simulink model "sampleModel1516"  (R2023a)
settings: Solver=VariableStepAuto  StartTime=0.0  StopTime=10.0  RelTol=1e-3
libraries: hdlsllib x5, simulink x1
settings Model: Creator=user1  LastModifiedBy=user1

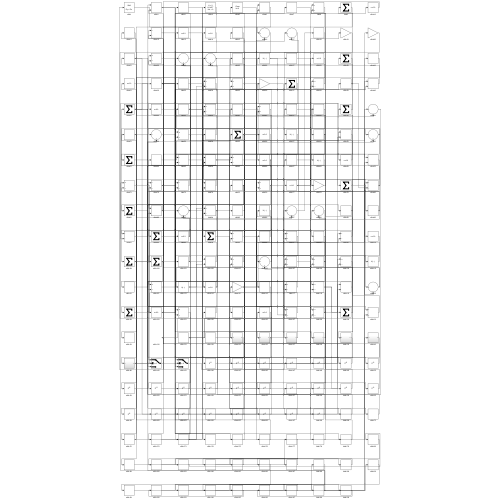
[thumbnail: Simulink's stored preview of the top-level diagram]
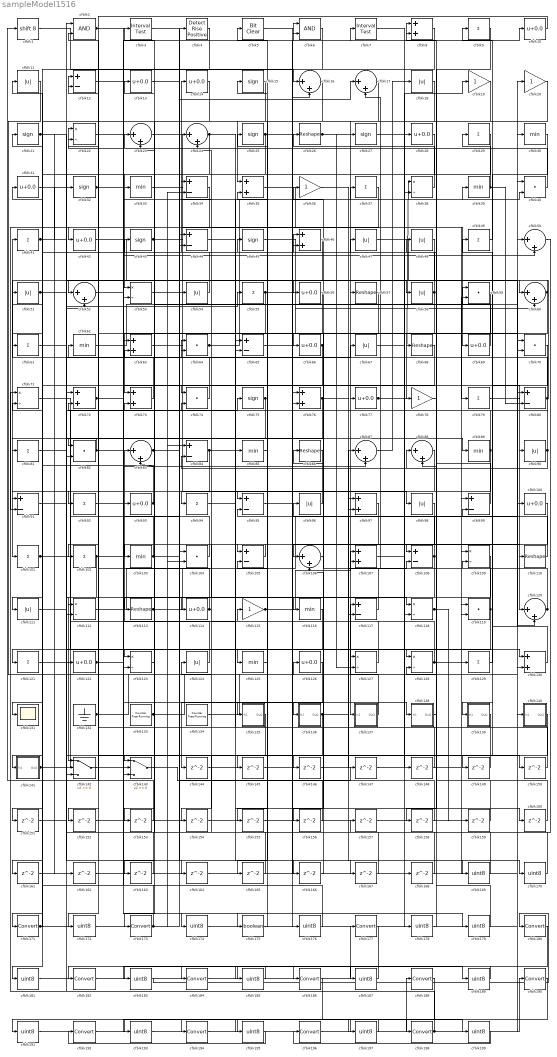
== system sampleModel1516 ==
  cfblk1 : ArithShift  BitShiftNumber=8
  cfblk{10,13..14,28,31,42,56,66,69,77,93,100,114,122,126} (15 alike) : Bias  Bias=0.0  SaturateOnIntegerOverflow=off
  cfblk{9,29,37,41,49,55,61,79,81,92,94,101..102,121,129} (15 alike) : Sum  Inputs=+
  cfblk{30,33,39,62,85,89,103,116,125} (9 alike) : MinMax
  cfblk{40,59,64,70,74,82,104,119} (8 alike) : DotProduct  OutDataTypeStr=Inherit: Inherit via internal rule
  cfblk{12,34,44,65,80,84,91,95,99,105,108,117} (12 alike) : Sum  Inputs=+-
  cfblk{16..17,23..24,50,52,60,83,87..88,106,120} (12 alike) : Sum  Inputs=|++
  cfblk{8,35,46,63,72..73,76,97,107,130} (10 alike) : Sum
  cfblk{22,38,53,71,109,112,118,123,127..128} (10 alike) : Product  Inputs=*/  RndMeth=Zero  SaturateOnIntegerOverflow=on
  cfblk{11,18,47..48,51,54,58,67,90,96,98,111,124} (13 alike) : Abs  SaturateOnIntegerOverflow=off
  cfblk{26,57,68,86,110,113} (6 alike) : Reshape
  cfblk{19..20,36,78,115} (5 alike) : Gain
  cfblk131 : Scope
  cfblk132 : Ground
  cfblk133 : hdlsllib/Sources/Counter Free-Running  NumBits=16  tsamp=-1
  cfblk134 : hdlsllib/Sources/Counter Free-Running  NumBits=16  tsamp=-1
  cfblk135 : Subsystem
      settings: LibrarySourceBlock=|
      | hdlsllib/Ports &
      | Subsystems/Subsystem
  cfblk136 : Subsystem
      settings: LibrarySourceBlock=|
      | hdlsllib/Ports &
      | Subsystems/Subsystem
  cfblk137 : Subsystem
      settings: LibrarySourceBlock=|
      | hdlsllib/Ports &
      | Subsystems/Subsystem
  cfblk138 : Subsystem
      settings: LibrarySourceBlock=|
      | hdlsllib/Ports &
      | Subsystems/Subsystem
  cfblk139 : Subsystem
      settings: LibrarySourceBlock=|
      | hdlsllib/Ports &
      | Subsystems/Subsystem
  cfblk140 : Subsystem
      settings: LibrarySourceBlock=|
      | hdlsllib/Ports &
      | Subsystems/Subsystem
  cfblk141 : Subsystem
      settings: LibrarySourceBlock=|
      | hdlsllib/Ports &
      | Subsystems/Subsystem
  cfblk142 : Switch  SaturateOnIntegerOverflow=off  InputSameDT=off
  cfblk143 : Switch  SaturateOnIntegerOverflow=off  InputSameDT=off
  cfblk{144..168} (25 alike) : Delay  SampleTime=1
  cfblk{15,21,25,27,32,43,45,75} (8 alike) : Signum
  cfblk{169..170,172,174,176,178..179,181,183,185,187,189,191,193,195,197,199} (17 alike) : DataTypeConversion  OutDataTypeStr=uint8  SaturateOnIntegerOverflow=off  RndMeth=Floor
  cfblk{171,173,177,180,182,184,186,188,190,192,194,196,198} (13 alike) : DataTypeConversion  SaturateOnIntegerOverflow=off  RndMeth=Floor
  cfblk175 : DataTypeConversion  OutDataTypeStr=boolean  SaturateOnIntegerOverflow=off  RndMeth=Floor
  cfblk2 : Logic  AllPortsSameDT=off  OutDataTypeStr=boolean
  cfblk3 : hdlsllib/Logic and Bit Operations/Interval Test  IntervalClosedRight=on  uplimit=0.5  IntervalClosedLeft=on  lowlimit=-0.5  OutDataTypeStr=boolean
  cfblk4 : hdlsllib/Logic and Bit Operations/Detect Rise Positive  vinit=0  OutDataTypeStr=boolean
  cfblk5 : simulink/Logic and Bit Operations/Bit Clear  iBit=0
      settings: LibrarySourceBlock=|
      | hdlsllib/Logic and Bit
      | Operations/Bit Clear
  cfblk6 : Logic  AllPortsSameDT=off  OutDataTypeStr=boolean
  cfblk7 : hdlsllib/Logic and Bit Operations/Interval Test  IntervalClosedRight=on  uplimit=0.5  IntervalClosedLeft=on  lowlimit=-0.5  OutDataTypeStr=boolean
  wires:
  cfblk41/1 -> cfblk32/1, cfblk56/1, cfblk164/1
  cfblk87/1 -> cfblk18/1
  cfblk77/1 -> cfblk38/1, cfblk19/1
  cfblk46/1 -> cfblk101/1
  cfblk8/1 -> cfblk16/1
  cfblk58/1 -> cfblk14/1, cfblk97/2, cfblk153/1
  cfblk74/1 -> cfblk41/1
  cfblk29/1 -> cfblk53/1
  cfblk19/1 -> cfblk35/1
  cfblk30/1 -> cfblk143/1
  cfblk110/1 -> cfblk96/1
  cfblk85/1 -> cfblk15/1
  cfblk124/1 -> cfblk83/1
  cfblk79/1 -> cfblk120/1
  cfblk53/1 -> cfblk66/1
  cfblk20/1 -> cfblk137/1(In1)
  cfblk118/1 -> cfblk129/1, cfblk159/1
  cfblk42/1 -> cfblk58/1
  cfblk11/1 -> cfblk126/1
  cfblk60/1 -> cfblk73/1, cfblk57/1
  cfblk105/1 -> cfblk103/1
  cfblk139/1(Out1) -> cfblk125/1
  cfblk96/1 -> cfblk95/1
  cfblk80/1 -> cfblk60/1, cfblk72/2, cfblk23/2
  cfblk75/1 -> cfblk121/1, cfblk102/1
  cfblk55/1 -> cfblk60/2, cfblk122/1, cfblk108/1
  cfblk54/1 -> cfblk31/1
  cfblk128/1 -> cfblk119/1, cfblk64/2
  cfblk141/1(Out1) -> cfblk75/1, cfblk52/2
  cfblk106/1 -> cfblk46/1
  cfblk109/1 -> cfblk142/1
  cfblk66/1 -> cfblk111/1, cfblk135/1(In1)
  cfblk137/1(Out1) -> cfblk117/1
  cfblk23/1 -> cfblk98/1
  cfblk102/1 -> cfblk33/1, cfblk112/2
  cfblk10/1 -> cfblk42/1
  cfblk35/1 -> cfblk69/1
  cfblk16/1 -> cfblk61/1
  cfblk97/1 -> cfblk136/1(In1)
  cfblk115/1 -> cfblk107/1, cfblk99/2
  cfblk47/1 -> cfblk70/1
  cfblk64/1 -> cfblk20/1, cfblk166/1
  cfblk112/1 -> cfblk50/1
  cfblk119/1 -> cfblk47/1, cfblk143/3
  cfblk71/1 -> cfblk130/1
  cfblk140/1(Out1) -> cfblk173/1
  cfblk68/1 -> cfblk116/1
  cfblk86/1 -> cfblk92/1
  cfblk72/1 -> cfblk74/1, cfblk117/2
  cfblk40/1 -> cfblk22/1
  cfblk91/1 -> cfblk67/1
  cfblk31/1 -> cfblk123/1
  cfblk38/1 -> cfblk26/1
  cfblk125/1 -> cfblk45/1
  cfblk14/1 -> cfblk53/2
  cfblk69/1 -> cfblk13/1
  cfblk82/1 -> cfblk81/1, cfblk179/1
  cfblk39/1 -> cfblk29/1, cfblk80/2
  cfblk122/1 -> cfblk6/1, cfblk40/2
  cfblk13/1 -> cfblk104/1
  cfblk78/1 -> cfblk8/1
  cfblk65/1 -> cfblk127/1
  cfblk70/1 -> cfblk139/1(In1)
  cfblk17/1 -> cfblk112/1
  cfblk108/1 -> cfblk35/2, cfblk156/1
  cfblk121/1 -> cfblk85/1
  cfblk132/1 -> cfblk1/1, cfblk24/1
  cfblk99/1 -> cfblk62/1
  cfblk44/1 -> cfblk77/1
  cfblk93/1 -> cfblk51/1, cfblk83/2
  cfblk62/1 -> cfblk40/1
  cfblk25/1 -> cfblk68/1, cfblk161/1
  cfblk12/1 -> cfblk87/2
  cfblk15/1 -> cfblk113/1
  cfblk89/1 -> cfblk94/1, cfblk25/1
  cfblk103/1 -> cfblk59/1, cfblk93/1
  cfblk73/1 -> cfblk11/1
  cfblk43/1 -> cfblk120/2, cfblk17/1
  cfblk116/1 -> cfblk131/1
  cfblk117/1 -> cfblk86/1
  cfblk26/1 -> cfblk27/1, cfblk127/2
  cfblk134/1 -> cfblk70/2
  cfblk51/1 -> cfblk91/1, cfblk123/2
  cfblk83/1 -> cfblk6/2, cfblk43/1
  cfblk138/1(Out1) -> cfblk48/1
  cfblk59/1 -> cfblk106/1
  cfblk34/1 -> cfblk91/2
  cfblk130/1 -> cfblk109/2
  cfblk101/1 -> cfblk44/2, cfblk63/2
  cfblk129/1 -> cfblk49/1
  cfblk32/1 -> cfblk10/1, cfblk50/2, cfblk118/1, cfblk138/1(In1)
  cfblk111/1 -> cfblk73/2
  cfblk4/1 -> cfblk171/1
  cfblk28/1 -> cfblk63/1
  cfblk104/1 -> cfblk23/1
  cfblk127/1 -> cfblk115/1
  cfblk84/1 -> cfblk34/1, cfblk37/1, cfblk151/1
  cfblk63/1 -> cfblk90/1
  cfblk37/1 -> cfblk52/1
  cfblk133/1 -> cfblk97/1, cfblk28/1
  cfblk27/1 -> cfblk78/1
  cfblk114/1 -> cfblk12/1, cfblk24/2
  cfblk6/1 -> cfblk82/1
  cfblk21/1 -> cfblk89/1, cfblk162/1
  cfblk49/1 -> cfblk9/1
  cfblk142/1 -> cfblk39/1
  cfblk76/1 -> cfblk110/1, cfblk142/3
  cfblk136/1(Out1) -> cfblk108/2, cfblk154/1
  cfblk95/1 -> cfblk128/1
  cfblk113/1 -> cfblk7/1, cfblk104/2
  cfblk120/1 -> cfblk107/2, cfblk64/1
  cfblk100/1 -> cfblk114/1
  cfblk1/1 -> cfblk76/2
  cfblk90/1 -> cfblk36/1, cfblk84/2, cfblk17/2
  cfblk18/1 -> cfblk105/1
  cfblk45/1 -> cfblk100/1
  cfblk2/1 -> cfblk65/2, cfblk118/2
  cfblk61/1 -> cfblk55/1
  cfblk33/1 -> cfblk79/1
  cfblk24/1 -> cfblk141/1(In1), cfblk167/1
  cfblk126/1 -> cfblk144/1
  cfblk144/1 -> cfblk119/2
  cfblk57/1 -> cfblk145/1
  cfblk145/1 -> cfblk87/1
  cfblk81/1 -> cfblk146/1
  cfblk146/1 -> cfblk59/2
  cfblk143/1 -> cfblk147/1
  cfblk147/1 -> cfblk38/2
  cfblk107/1 -> cfblk148/1
  cfblk148/1 -> cfblk65/1
  cfblk67/1 -> cfblk149/1
  cfblk149/1 -> cfblk12/2
  cfblk52/1 -> cfblk150/1
  cfblk150/1 -> cfblk22/2
  cfblk151/1 -> cfblk82/2
  cfblk135/1(Out1) -> cfblk152/1
  cfblk152/1 -> cfblk16/2
  cfblk153/1 -> cfblk2/2
  cfblk154/1 -> cfblk74/2
  cfblk98/1 -> cfblk155/1
  cfblk155/1 -> cfblk109/1
  cfblk156/1 -> cfblk105/2
  cfblk50/1 -> cfblk157/1
  cfblk9/1 -> cfblk158/1
  cfblk158/1 -> cfblk44/1
  cfblk159/1 -> cfblk128/2
  cfblk94/1 -> cfblk160/1
  cfblk160/1 -> cfblk8/2
  cfblk161/1 -> cfblk46/2
  cfblk162/1 -> cfblk99/1
  cfblk123/1 -> cfblk163/1
  cfblk163/1 -> cfblk72/1
  cfblk164/1 -> cfblk80/1
  cfblk56/1 -> cfblk165/1
  cfblk165/1 -> cfblk142/2
  cfblk166/1 -> cfblk106/2
  cfblk167/1 -> cfblk95/2
  cfblk7/1 -> cfblk168/1
  cfblk168/1 -> cfblk76/1
  cfblk3/1 -> cfblk169/1
  cfblk169/1 -> cfblk124/1
  cfblk36/1 -> cfblk170/1
  cfblk170/1 -> cfblk3/1
  cfblk171/1 -> cfblk54/1, cfblk21/1
  cfblk48/1 -> cfblk172/1
  cfblk172/1 -> cfblk4/1
  cfblk173/1 -> cfblk71/2, cfblk34/2, cfblk84/1
  cfblk22/1 -> cfblk174/1
  cfblk174/1 -> cfblk140/1(In1)
  cfblk92/1 -> cfblk175/1
  cfblk175/1 -> cfblk5/1
  cfblk5/1 -> cfblk176/1
  cfblk176/1 -> cfblk143/2
  cfblk157/1 -> cfblk178/1
  cfblk178/1 -> cfblk88/1
  cfblk179/1 -> cfblk88/2
  cfblk88/1 -> cfblk181/1
  cfblk181/1 -> cfblk177/1
  cfblk177/1 -> cfblk183/1
  cfblk183/1 -> cfblk180/1
  cfblk180/1 -> cfblk185/1
  cfblk185/1 -> cfblk182/1
  cfblk182/1 -> cfblk187/1
  cfblk187/1 -> cfblk184/1
  cfblk184/1 -> cfblk189/1
  cfblk189/1 -> cfblk186/1
  cfblk186/1 -> cfblk191/1
  cfblk191/1 -> cfblk188/1
  cfblk188/1 -> cfblk193/1
  cfblk193/1 -> cfblk190/1
  cfblk190/1 -> cfblk195/1
  cfblk195/1 -> cfblk192/1
  cfblk196/1 -> cfblk198/1
  cfblk192/1 -> cfblk197/1
  cfblk197/1 -> cfblk194/1
  cfblk198/1 -> cfblk130/2, cfblk71/1, cfblk2/1, cfblk30/1
  cfblk194/1 -> cfblk199/1
  cfblk199/1 -> cfblk196/1

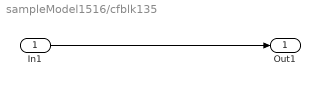
== system sampleModel1516/cfblk135 ==
  In1 : Inport
  Out1 : Outport
  wires:
  In1/1 -> Out1/1

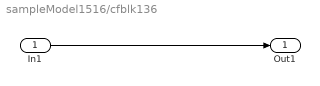
== system sampleModel1516/cfblk136 ==
  In1 : Inport
  Out1 : Outport
  wires:
  In1/1 -> Out1/1

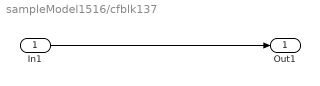
== system sampleModel1516/cfblk137 ==
  In1 : Inport
  Out1 : Outport
  wires:
  In1/1 -> Out1/1

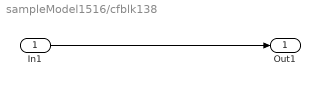
== system sampleModel1516/cfblk138 ==
  In1 : Inport
  Out1 : Outport
  wires:
  In1/1 -> Out1/1

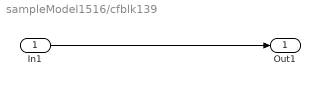
== system sampleModel1516/cfblk139 ==
  In1 : Inport
  Out1 : Outport
  wires:
  In1/1 -> Out1/1

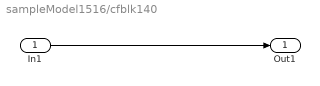
== system sampleModel1516/cfblk140 ==
  In1 : Inport
  Out1 : Outport
  wires:
  In1/1 -> Out1/1

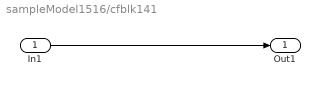
== system sampleModel1516/cfblk141 ==
  In1 : Inport
  Out1 : Outport
  wires:
  In1/1 -> Out1/1
